simulink model "testFTSensorsLegs"  (Simulink 8.6)
settings: Solver=FixedStepDiscrete  StartTime=0.0  StopTime=inf  FixedStep=0.01  RelTol=1e-3
InitFcn:
  | initRefGen;
libraries: WBToolboxLibrary x7, WBCLibrary x1
settings Model: Creator=DanielePucci  LastModifiedBy=DanielePucci
settings DataIOCC: SaveFormat=Dataset  SignalLoggingSaveFormat=Dataset
settings OptimizationCC: ExpressionDepthLimit=128
settings DebuggingCC: UnderspecifiedInitializationDetection=Simplified  MergeDetectMultiDrivingBlocksExec=error  SolverPrmCheckMsg=none  FcnCallInpInsideContextMsg=EnableAllAsError  StateNameClashWarn=none
settings HardwareCC: ProdBitPerPointer=64  ProdLargestAtomicFloat=Float  ProdIntDivRoundTo=Zero  ProdEndianess=LittleEndian  ProdWordSize=64  ProdHWDeviceType=Intel->x86-64 (Windows64)
settings GRTTargetCC: GeneratePreprocessorConditionals=Use local settings  CombineOutputUpdateFcns=on  GRTInterface=off
settings ConfigComp: CovModelRefEnable=off

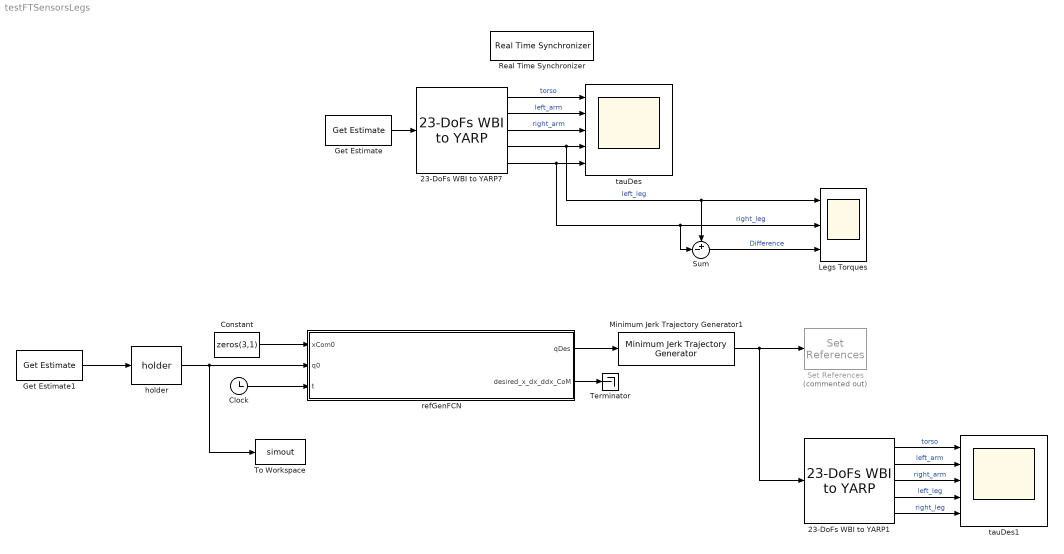
== system testFTSensorsLegs ==
  23-DoFs WBI to YARP1 : WBToolboxLibrary/Utilities/23-DoFs WBI to YARP
  23-DoFs WBI to YARP7 : WBToolboxLibrary/Utilities/23-DoFs WBI to YARP
  Clock : Clock
  Constant : Constant  Value=zeros(3,1)
  Get Estimate : WBToolboxLibrary/wholeBodyStates/Get Estimate  estimateType=Joints Torque  robotName=WBT_robotName  localName=WBT_modelName  wbiFile=WBT_wbiFilename  wbiList=WBT_wbiList
  Get Estimate1 : WBToolboxLibrary/wholeBodyStates/Get Estimate  estimateType=Joints Position  robotName=WBT_robotName  localName=WBT_modelName  wbiFile=WBT_wbiFilename  wbiList=WBT_wbiList
  Legs Torques : Scope  NumInputPorts=3
  Minimum Jerk Trajectory Generator1 : WBToolboxLibrary/Utilities/Minimum Jerk Trajectory Generator  externalSettlingTime=off  settlingTime=references.joints.smoothingTime  sampleTime=CONFIG.Ts  firstDerivatives=off  secondDerivatives=off  explicitInitialValue=off
  Real Time Synchronizer : WBCLibrary/Utilities/Real Time Synchronizer  Priority=-10  threadPeriod=0.01
  Set References : WBToolboxLibrary/wholeBodyActuators/Set References  Commented=on  controlType=Position Direct  robotName=WBT_robotName  localName=WBT_modelName  wbiFile=WBT_wbiFilename  wbiList=WBT_wbiList
  Sum : Sum  Inputs=+-|
  Terminator : Terminator
  To Workspace : ToWorkspace  VariableName=simout  SaveFormat=Timeseries  SampleTime=-1
  "holder " : WBToolboxLibrary/Utilities/holder 
  refGenFCN : MATLAB Function  TreatAsAtomicUnit=on
  tauDes : Scope  NumInputPorts=5
  tauDes1 : Scope  NumInputPorts=5
  wires:
  23-DoFs WBI to YARP7/5 -> Legs Torques/2, Sum/2, tauDes/5  "right_leg"
  23-DoFs WBI to YARP7/1 -> tauDes/1  "torso"
  23-DoFs WBI to YARP7/2 -> tauDes/2  "left_arm"
  23-DoFs WBI to YARP7/4 -> Sum/1, Legs Torques/1, tauDes/4  "left_leg"
  23-DoFs WBI to YARP7/3 -> tauDes/3  "right_arm"
  Get Estimate/1 -> 23-DoFs WBI to YARP7/1
  refGenFCN/2(desired_x_dx_ddx_CoM) -> Terminator/1
  Clock/1 -> refGenFCN/3(t)
  Get Estimate1/1 -> "holder "/1
  "holder "/1 -> To Workspace/1, refGenFCN/2(q0)
  Constant/1 -> refGenFCN/1(xCom0)
  refGenFCN/1(qDes) -> Minimum Jerk Trajectory Generator1/1
  23-DoFs WBI to YARP1/5 -> tauDes1/5  "right_leg"
  23-DoFs WBI to YARP1/1 -> tauDes1/1  "torso"
  23-DoFs WBI to YARP1/2 -> tauDes1/2  "left_arm"
  23-DoFs WBI to YARP1/4 -> tauDes1/4  "left_leg"
  23-DoFs WBI to YARP1/3 -> tauDes1/3  "right_arm"
  Minimum Jerk Trajectory Generator1/1 -> 23-DoFs WBI to YARP1/1, Set References/1
  Sum/1 -> Legs Torques/3  "Difference"

== matlab function refGenFCN ==
  data: xCom0 input double; qDes output double; q0 input double; t input double; references parameter double; desired_x_dx_ddx_CoM output double
function [qDes,desired_x_dx_ddx_CoM] = refGenFCN(xCom0,q0,t,references)
%#codegen

[qDes,desired_x_dx_ddx_CoM] = refGen(xCom0,q0,t,references);
